simulink model "eg_5_03_R2018a"  (R2018a)
settings: Solver=ode4  StartTime=0.0  StopTime=10  FixedStep=0.001  RelTol=1e-3  EnableMultiTasking=on
values from neighbouring files (symbols this model uses):
  A = [ 0  1  0  0 ... (first row only)    [eg_5_01a.m]    (also in eg_5_01b.m; eg_5_01c.m; eg_5_01d.m; eg_5_02.m = [ -2  1)
  b = [ 0 ... (first row only)    [eg_5_01a.m]    (also in eg_5_01b.m; eg_5_01c.m; eg_5_01d.m; eg_5_02.m = [  0)
  c = [ 0  0  1  0 ]    [eg_5_01a.m]    (also in eg_5_01b.m; eg_5_01c.m; eg_5_01d.m; eg_5_02.m = [ -2  2 ])
  h = [ -k  1 ]*inv(M0)*[ zeros(4,1) ... (first row only)    [eg_5_01b.m]    (also in eg_5_01c.m; eg_5_01d.m = 10; eg_5_03a.m = 10; eg_5_03b.m = 10)
  k = - e*inv(Vc)*Delta_A    [eg_5_01b.m]    (also in eg_5_01c.m = - acker(A,b,p); eg_5_01d.m = [ -7/2 -5/2 -13/2 -11/2]; eg_5_03a.m = [ -7/2 -5/2 -13/2 -11/2]; eg_5_03b.m = [ -7/2 -5/2 -13/2 -11/2])
settings Model: Creator=kawata  LastModifiedBy=kawata
settings DataIOCC: LimitDataPoints=on  SaveFormat=Array  SignalLoggingSaveFormat=ModelDataLogs  SignalLoggingName=sigsOut
settings OptimizationCC: ExpressionDepthLimit=2147483647  LifeSpan=inf
settings DebuggingCC: SaveWithParameterizedLinksMsg=none  UnderspecifiedInitializationDetection=Classic  MergeDetectMultiDrivingBlocksExec=none  SignalResolutionControl=TryResolveAllWithWarning  MultiTaskDSMMsg=warning  MultiTaskCondExecSysMsg=none  FcnCallInpInsideContextMsg=warning  StateNameClashWarn=warning  SFUnexpectedBacktrackingDiag=warning  SFNoUnconditionalDefaultTransitionDiag=warning  SFExecutionAtInitializationDiag=none
settings HardwareCC: ProdBitPerPointer=32  ProdBitPerSizeT=32  ProdBitPerPtrDiffT=32  ProdLargestAtomicFloat=None  ProdIntDivRoundTo=Undefined  ProdEndianess=Unspecified  ProdWordSize=32  ProdHWDeviceType=32-bit Generic  TargetUnknown=on
settings ModelReferenceCC: PropagateSignalLabelsOutOfModel=off
settings CodeAppCC: StateflowObjectComments=on
settings GRTTargetCC: TargetLangStandard=C89/C90 (ANSI)  GeneratePreprocessorConditionals=Disable all  CombineOutputUpdateFcns=off  GRTInterface=on
settings ConfigComp: CovMetricSettings=dw  CovHtmlReporting=on  CovSaveCumulativeToWorkspaceVar=on  CovSaveSingleToWorkspaceVar=on  CovExternalEMLEnable=off

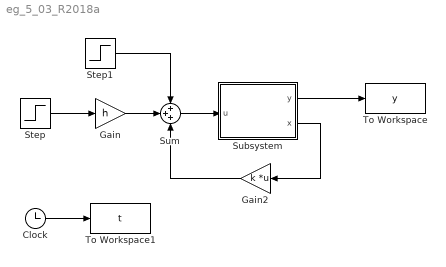
== system eg_5_03_R2018a ==
  Clock : Clock
  Gain : Gain  Gain=h  SaturateOnIntegerOverflow=on  OutDataTypeStr=Inherit: Same as input  ParamDataTypeStr=Inherit: Same as input
  Gain2 : Gain  Gain=k  Multiplication=Matrix(K*u)  SaturateOnIntegerOverflow=on  OutDataTypeStr=Inherit: Same as input  ParamDataTypeStr=Inherit: Same as input
  Step : Step  Time=0  SampleTime=0
  Step1 : Step  Time=5  SampleTime=0
  Subsystem : Subsystem
  Sum : Sum  Inputs=+++  SaturateOnIntegerOverflow=on  InputSameDT=on  OutDataTypeStr=Inherit: Same as first input
  To Workspace : ToWorkspace  VariableName=y  SampleTime=-1
  To Workspace1 : ToWorkspace  VariableName=t  SampleTime=-1
  wires:
  Subsystem/1(y) -> To Workspace/1
  Subsystem/2(x) -> Gain2/1
  Step/1 -> Gain/1
  Sum/1 -> Subsystem/1(u)
  Clock/1 -> To Workspace1/1
  Step1/1 -> Sum/1
  Gain/1 -> Sum/2
  Gain2/1 -> Sum/3

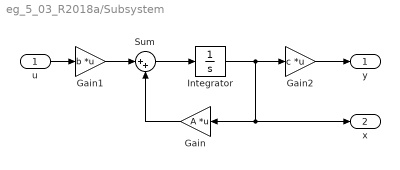
== system eg_5_03_R2018a/Subsystem ==
  u : Inport
  Gain : Gain  Gain=A  Multiplication=Matrix(K*u)  SaturateOnIntegerOverflow=on  OutDataTypeStr=Inherit: Same as input  ParamDataTypeStr=Inherit: Same as input
  Gain1 : Gain  Gain=b  Multiplication=Matrix(K*u)  SaturateOnIntegerOverflow=on  OutDataTypeStr=Inherit: Same as input  ParamDataTypeStr=Inherit: Same as input
  Gain2 : Gain  Gain=c  Multiplication=Matrix(K*u)  SaturateOnIntegerOverflow=on  OutDataTypeStr=Inherit: Same as input  ParamDataTypeStr=Inherit: Same as input
  Integrator : Integrator
  Sum : Sum  Inputs=|++  SaturateOnIntegerOverflow=on  InputSameDT=on  OutDataTypeStr=Inherit: Same as first input
  y : Outport
  x : Outport  Port=2
  wires:
  Gain/1 -> Sum/2
  Sum/1 -> Integrator/1
  Gain1/1 -> Sum/1
  Integrator/1 -> Gain2/1, Gain/1, x/1
  u/1 -> Gain1/1
  Gain2/1 -> y/1
